simulink model "Powertrain_model_21a"  (R2021a)
settings: Solver=VariableStepAuto  StartTime=0.0  StopTime=1000  RelTol=1e-3
values from neighbouring files (symbols this model uses):
  DR = 5.213    [Sim_script.m]    (also in workspace.mat)
  MaxLimit = [2.1951    294.39 ... (first row only)    [power_distribute_func.m]
  P_CE_idle = 0    [Sim_script.m]    (also in workspace.mat = 1)
  Trans_In = 24.086    [Sim_script.m]    (also in workspace.mat)
  w_CE_idle = 400    [Sim_script.m]    (also in workspace.mat = 32)
undefined symbols (not defined in the file or in its folder): Fuel_con_map, Res_Torque
libraries: pid_lib x2
settings Model: Creator=Sagar Singhal  LastModifiedBy=olsonsao

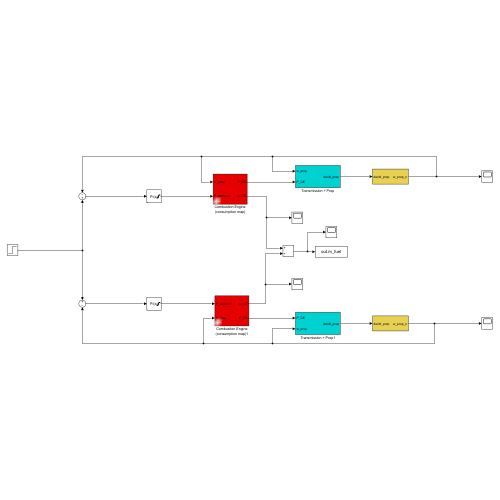
[thumbnail: Simulink's stored preview of the top-level diagram]
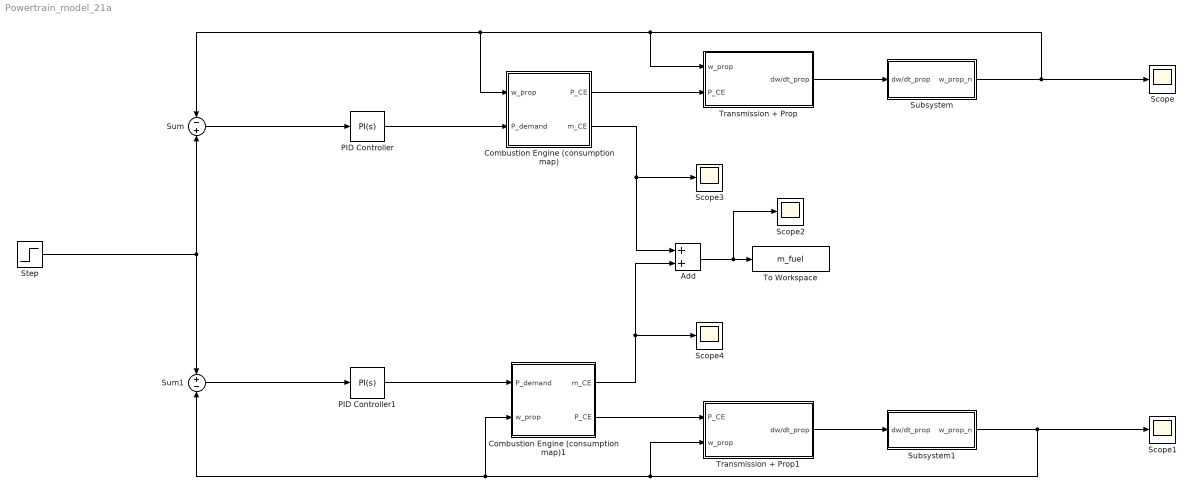
== system Powertrain_model_21a ==
  Add : Sum
  Combustion Engine (consumption map) : Subsystem  Tag=combustion engine  AncestorBlock=|
      | qss_tb_library/Energy Converter/Combustion Engine
      | (consumption map)
  Combustion Engine (consumption map)1 : Subsystem  Tag=combustion engine  AncestorBlock=|
      | qss_tb_library/Energy Converter/Combustion Engine
      | (consumption map)
  PID Controller : pid_lib/PID Controller  Controller=PI  Form=Parallel  TimeDomain=Continuous-time  UseExternalTs=off  SampleTime=-1  IntegratorMethod=Forward Euler  FilterMethod=Forward Euler  ControllerParametersSource=internal  P=6.64458766097002  I=6.35561266010105  D=0  UseFilter=on  N=100  TunerSelectOption=Transfer Function Based (PID Tuner App)  InitialConditionSource=internal  InitialConditionForIntegrator=0  InitialConditionForFilter=0  DifferentiatorICPrevScaledInput=0  ExternalReset=none  TrackingMode=off  Kt=1  LimitOutput=on  SatLimitsSource=internal  UpperSaturationLimit=inf  LowerSaturationLimit=0  LinearizeAsGain=on  AntiWindupMode=none  Kb=1  POutMin=[]  POutMax=[]  IOutMin=[]  IOutMax=[]  DOutMin=[]  DOutMax=[]  NOutMin=[]  NOutMax=[]  SumOutMin=[]  SumOutMax=[]  SaturationOutMin=[]  SaturationOutMax=[]  PParamMin=[]  PParamMax=[]  IParamMin=[]  IParamMax=[]  DParamMin=[]  DParamMax=[]  NParamMin=[]  NParamMax=[]  KbParamMin=[]  KbParamMax=[]  KtParamMin=[]  KtParamMax=[]  KbOutMin=[]  KbOutMax=[]  KtOutMin=[]  KtOutMax=[]  IntegratorOutMin=[]  IntegratorOutMax=[]  FilterOutMin=[]  FilterOutMax=[]  SumI1OutMin=[]  SumI1OutMax=[]  SumI2OutMin=[]  SumI2OutMax=[]  SumI3OutMin=[]  SumI3OutMax=[]  SumI4OutMin=[]  SumI4OutMax=[]  SumDOutMin=[]  SumDOutMax=[]  DifferentiatorOutMin=[]  DifferentiatorOutMax=[]  FilterDiffOutCoefMin=[]  FilterDiffOutCoefMax=[]  ReciprocalOutMin=[]  ReciprocalOutMax=[]  SumDenOutMin=[]  SumDenOutMax=[]  SumNumOutMin=[]  SumNumOutMax=[]  DivideOutMin=[]  DivideOutMax=[]  UdiffTsProdOutMin=[]  UdiffTsProdOutMax=[]  NTsProdOutMin=[]  NTsProdOutMax=[]  UintegralTsProdOutMin=[]  UintegralTsProdOutMax=[]  UngainTsProdOutMin=[]  UngainTsProdOutMax=[]  IntegratorContinuousStateAttributes=''  IntegratorStateMustResolveToSignalObject=off  IntegratorRTWStateStorageClass=Auto  FilterContinuousStateAttributes=''  FilterStateMustResolveToSignalObject=off  FilterRTWStateStorageClass=Auto  ParallelPVariant=InternalParameters  IdealPVariant=Disabled  IVariant=InternalParameters  DVariant=Disabled  IntegratorVariant=Continuous  SatVariant=Enabled  AWVariant=Passthrough  PCopyVariant=Disabled  TRVariant=Disabled  FdbkBlocksVariant=Forward  IdealPFdbkVariant=Disabled  SatFdbkVariant=Disabled  DerivativeFilterVariant=Disabled  NVariant=Disabled  NCopyVariant=Disabled_SignalSpec  FilterICVariant=Disabled  IntegratorICVariant=InternalICs  ExternalResetVariant=Disabled  TRSumVariant=Passthrough  SumFdbkVariant=Disabled  SumVariant=Sum_PI  TsampFilterVariant=InternalTs  TsampNgainVariant=Passthrough  TsampIntegralVariant=Passthrough  ExternalSaturationOutDataTypeStr=Inherit: Same as second input
  PID Controller1 : pid_lib/PID Controller  Controller=PI  Form=Parallel  TimeDomain=Continuous-time  UseExternalTs=off  SampleTime=-1  IntegratorMethod=Forward Euler  FilterMethod=Forward Euler  ControllerParametersSource=internal  P=6.64458766097002  I=6.35561266010105  D=0  UseFilter=on  N=100  TunerSelectOption=Transfer Function Based (PID Tuner App)  InitialConditionSource=internal  InitialConditionForIntegrator=0  InitialConditionForFilter=0  DifferentiatorICPrevScaledInput=0  ExternalReset=none  TrackingMode=off  Kt=1  LimitOutput=on  SatLimitsSource=internal  UpperSaturationLimit=inf  LowerSaturationLimit=0  LinearizeAsGain=on  AntiWindupMode=none  Kb=1  POutMin=[]  POutMax=[]  IOutMin=[]  IOutMax=[]  DOutMin=[]  DOutMax=[]  NOutMin=[]  NOutMax=[]  SumOutMin=[]  SumOutMax=[]  SaturationOutMin=[]  SaturationOutMax=[]  PParamMin=[]  PParamMax=[]  IParamMin=[]  IParamMax=[]  DParamMin=[]  DParamMax=[]  NParamMin=[]  NParamMax=[]  KbParamMin=[]  KbParamMax=[]  KtParamMin=[]  KtParamMax=[]  KbOutMin=[]  KbOutMax=[]  KtOutMin=[]  KtOutMax=[]  IntegratorOutMin=[]  IntegratorOutMax=[]  FilterOutMin=[]  FilterOutMax=[]  SumI1OutMin=[]  SumI1OutMax=[]  SumI2OutMin=[]  SumI2OutMax=[]  SumI3OutMin=[]  SumI3OutMax=[]  SumI4OutMin=[]  SumI4OutMax=[]  SumDOutMin=[]  SumDOutMax=[]  DifferentiatorOutMin=[]  DifferentiatorOutMax=[]  FilterDiffOutCoefMin=[]  FilterDiffOutCoefMax=[]  ReciprocalOutMin=[]  ReciprocalOutMax=[]  SumDenOutMin=[]  SumDenOutMax=[]  SumNumOutMin=[]  SumNumOutMax=[]  DivideOutMin=[]  DivideOutMax=[]  UdiffTsProdOutMin=[]  UdiffTsProdOutMax=[]  NTsProdOutMin=[]  NTsProdOutMax=[]  UintegralTsProdOutMin=[]  UintegralTsProdOutMax=[]  UngainTsProdOutMin=[]  UngainTsProdOutMax=[]  IntegratorContinuousStateAttributes=''  IntegratorStateMustResolveToSignalObject=off  IntegratorRTWStateStorageClass=Auto  FilterContinuousStateAttributes=''  FilterStateMustResolveToSignalObject=off  FilterRTWStateStorageClass=Auto  ParallelPVariant=InternalParameters  IdealPVariant=Disabled  IVariant=InternalParameters  DVariant=Disabled  IntegratorVariant=Continuous  SatVariant=Enabled  AWVariant=Passthrough  PCopyVariant=Disabled  TRVariant=Disabled  FdbkBlocksVariant=Forward  IdealPFdbkVariant=Disabled  SatFdbkVariant=Disabled  DerivativeFilterVariant=Disabled  NVariant=Disabled  NCopyVariant=Disabled_SignalSpec  FilterICVariant=Disabled  IntegratorICVariant=InternalICs  ExternalResetVariant=Disabled  TRSumVariant=Passthrough  SumFdbkVariant=Disabled  SumVariant=Sum_PI  TsampFilterVariant=InternalTs  TsampNgainVariant=Passthrough  TsampIntegralVariant=Passthrough  ExternalSaturationOutDataTypeStr=Inherit: Same as second input
  Scope{,1..4} (5 alike) : Scope
  Step : Step  Time=500  Before=100  After=400  SampleTime=0
  Subsystem : Subsystem
  Subsystem1 : Subsystem
  Sum : Sum  Inputs=-|+
  Sum1 : Sum  Inputs=+|-
  To Workspace : ToWorkspace  VariableName=m_fuel  SaveFormat=Timeseries  SampleTime=-1
  Transmission + Prop : Subsystem
  Transmission + Prop1 : Subsystem
  wires:
  Combustion Engine (consumption map)/1(P_CE) -> Transmission + Prop/2(P_CE)
  Transmission + Prop/1(dw/dt_prop) -> Subsystem/1(dw/dt_prop)
  Combustion Engine (consumption map)/2(m_CE) -> Scope3/1, Add/1
  Subsystem/1(w_prop_n) -> Scope/1, Transmission + Prop/1(w_prop), Combustion Engine (consumption map)/1(w_prop), Sum/1
  Sum/1 -> PID Controller/1
  PID Controller/1 -> Combustion Engine (consumption map)/2(P_demand)
  PID Controller1/1 -> Combustion Engine (consumption map)1/1(P_demand)
  Sum1/1 -> PID Controller1/1
  Combustion Engine (consumption map)1/2(P_CE) -> Transmission + Prop1/1(P_CE)
  Subsystem1/1(w_prop_n) -> Scope1/1, Transmission + Prop1/2(w_prop), Sum1/2, Combustion Engine (consumption map)1/2(w_prop)
  Transmission + Prop1/1(dw/dt_prop) -> Subsystem1/1(dw/dt_prop)
  Combustion Engine (consumption map)1/1(m_CE) -> Scope4/1, Add/2
  Step/1 -> Sum/2, Sum1/1
  Add/1 -> To Workspace/1, Scope2/1

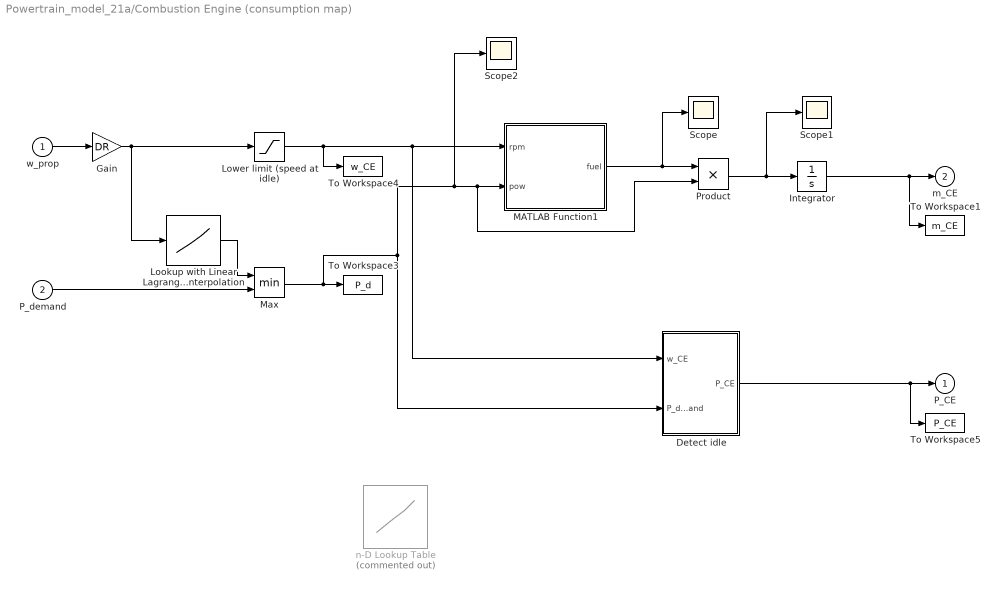
== system Powertrain_model_21a/Combustion Engine (consumption map) ==
  w_prop : Inport
  P_demand : Inport  Port=2
  Detect idle : Subsystem
  Gain : Gain  Gain=DR
  Integrator : Integrator
  Lookup with Linear Lagrange Interpolation : Lookup_n-D  NumberOfTableDimensions=1  BreakpointsForDimension1=MaxLimit.('RPM')  Table=MaxLimit.('Pow_kW_')  InterpMethod=Linear Lagrange  InternalRulePriority=Speed  RndMeth=Simplest  InputSameDT=on
  Lower limit (speed at idle) : Saturate  UpperLimit=inf  LowerLimit=w_CE_idle
  MATLAB Function1 : MATLAB Function  TreatAsAtomicUnit=on
  Max : MinMax  Inputs=2
  Product : Product
  Scope : Scope
  Scope1 : Scope
  Scope2 : Scope
  To Workspace1 : ToWorkspace  VariableName=m_CE  SampleTime=-1
  To Workspace3 : ToWorkspace  VariableName=P_d  SampleTime=-1
  To Workspace4 : ToWorkspace  VariableName=w_CE  SampleTime=-1
  To Workspace5 : ToWorkspace  VariableName=P_CE  SampleTime=-1
  n-D Lookup Table : Lookup_n-D  Commented=on  LookupTableObject=''  BreakpointsForDimension1=Fuel_con_map.('RPM')  BreakpointsForDimension2=Fuel_con_map.('Power(kW)')  BreakpointsForDimension3=[5, 7]  BreakpointsForDimension1FirstPoint=10  BreakpointsForDimension2FirstPoint=10  BreakpointsForDimension1Spacing=12  BreakpointsForDimension2Spacing=12  IndexSearchMethod=Evenly spaced points  Table=Fuel_con_map.('Fuel(g/KWh)')  InterpMethod=Cubic spline  ExtrapMethod=Cubic spline  DiagnosticForOutOfRangeInput=Error  InternalRulePriority=Speed  RndMeth=Simplest  InputSameDT=on
      settings: InputPortMap=u0,u1
  P_CE : Outport  InitialOutput=0
  m_CE : Outport  Port=2  InitialOutput=0
  wires:
  Integrator/1 -> To Workspace1/1, m_CE/1
  w_prop/1 -> Gain/1
  Detect idle/1(P_CE) -> To Workspace5/1, P_CE/1
  Lookup with Linear Lagrange Interpolation/1 -> Max/1
  Gain/1 -> Lookup with Linear Lagrange Interpolation/1, Lower limit (speed at idle)/1
  P_demand/1 -> Max/2
  MATLAB Function1/1(fuel) -> Scope/1, Product/1
  Lower limit (speed at idle)/1 -> To Workspace4/1, MATLAB Function1/1(rpm), Detect idle/1(w_CE)
  Product/1 -> Scope1/1, Integrator/1
  Max/1 -> Scope2/1, Product/2, MATLAB Function1/2(pow), Detect idle/2(P_demand), To Workspace3/1

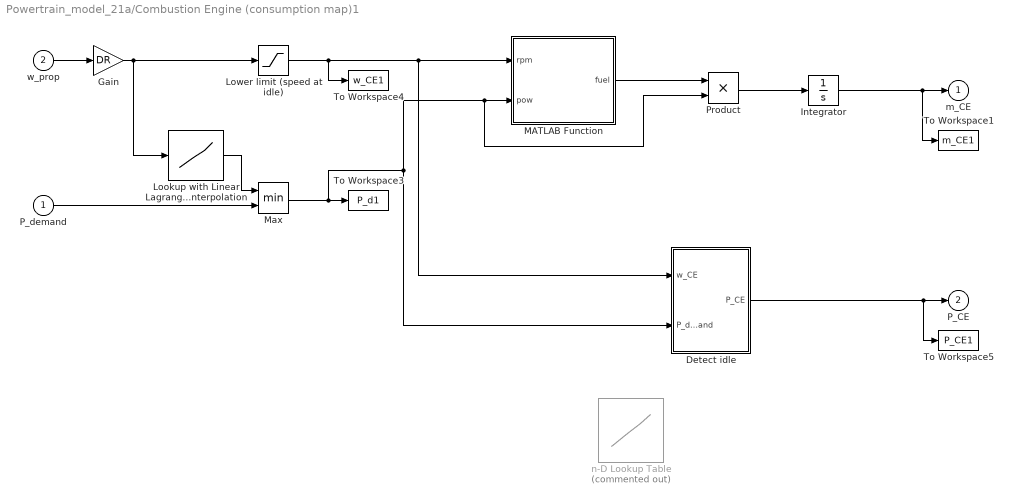
== system Powertrain_model_21a/Combustion Engine (consumption map)1 ==
  P_demand : Inport
  w_prop : Inport  Port=2
  Detect idle : Subsystem
  Gain : Gain  Gain=DR
  Integrator : Integrator
  Lookup with Linear Lagrange Interpolation : Lookup_n-D  NumberOfTableDimensions=1  BreakpointsForDimension1=MaxLimit.('RPM')  Table=MaxLimit.('Pow_kW_')  InterpMethod=Linear Lagrange  InternalRulePriority=Speed  RndMeth=Simplest  InputSameDT=on
  Lower limit (speed at idle) : Saturate  UpperLimit=inf  LowerLimit=w_CE_idle
  MATLAB Function : MATLAB Function  TreatAsAtomicUnit=on
  Max : MinMax  Inputs=2
  Product : Product
  To Workspace1 : ToWorkspace  VariableName=m_CE1  SampleTime=-1
  To Workspace3 : ToWorkspace  VariableName=P_d1  SampleTime=-1
  To Workspace4 : ToWorkspace  VariableName=w_CE1  SampleTime=-1
  To Workspace5 : ToWorkspace  VariableName=P_CE1  SampleTime=-1
  n-D Lookup Table : Lookup_n-D  Commented=on  LookupTableObject=''  BreakpointsForDimension1=Fuel_con_map.('RPM')  BreakpointsForDimension2=Fuel_con_map.('Power(kW)')  BreakpointsForDimension3=[5, 7]  BreakpointsForDimension1FirstPoint=10  BreakpointsForDimension2FirstPoint=10  BreakpointsForDimension1Spacing=12  BreakpointsForDimension2Spacing=12  IndexSearchMethod=Evenly spaced points  Table=Fuel_con_map.('Fuel(g/KWh)')  InterpMethod=Cubic spline  ExtrapMethod=Cubic spline  DiagnosticForOutOfRangeInput=Error  InternalRulePriority=Speed  RndMeth=Simplest  InputSameDT=on
      settings: InputPortMap=u0,u1
  m_CE : Outport  InitialOutput=0
  P_CE : Outport  Port=2  InitialOutput=0
  wires:
  Max/1 -> Product/2, MATLAB Function/2(pow), Detect idle/2(P_demand), To Workspace3/1
  Product/1 -> Integrator/1
  w_prop/1 -> Gain/1
  Lower limit (speed at idle)/1 -> To Workspace4/1, Detect idle/1(w_CE), MATLAB Function/1(rpm)
  Detect idle/1(P_CE) -> To Workspace5/1, P_CE/1
  Lookup with Linear Lagrange Interpolation/1 -> Max/1
  Gain/1 -> Lookup with Linear Lagrange Interpolation/1, Lower limit (speed at idle)/1
  P_demand/1 -> Max/2
  MATLAB Function/1(fuel) -> Product/1
  Integrator/1 -> To Workspace1/1, m_CE/1

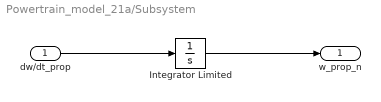
== system Powertrain_model_21a/Subsystem ==
  dw/dt_prop : Inport
  Integrator Limited : Integrator  InitialCondition=100  UpperSaturationLimit=1  LowerSaturationLimit=0
  w_prop_n : Outport
  wires:
  dw/dt_prop/1 -> Integrator Limited/1
  Integrator Limited/1 -> w_prop_n/1

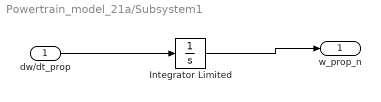
== system Powertrain_model_21a/Subsystem1 ==
  dw/dt_prop : Inport
  Integrator Limited : Integrator  InitialCondition=100  UpperSaturationLimit=1  LowerSaturationLimit=0
  w_prop_n : Outport
  wires:
  dw/dt_prop/1 -> Integrator Limited/1
  Integrator Limited/1 -> w_prop_n/1

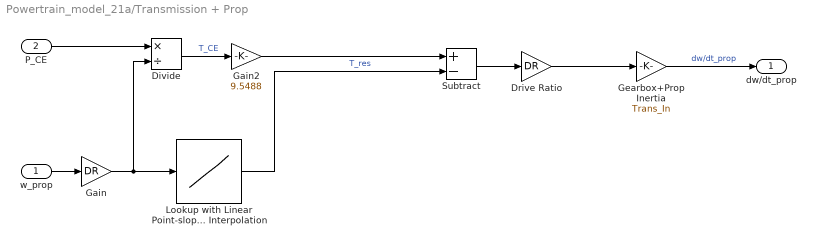
== system Powertrain_model_21a/Transmission + Prop ==
  w_prop : Inport
  P_CE : Inport  Port=2
  Divide : Product  Inputs=*/
  Drive Ratio : Gain  Gain=DR
  Gain : Gain  Gain=DR
  Gain2 : Gain  Gain=9.5488
  Gearbox+Prop Inertia : Gain  Gain=Trans_In
  Lookup with Linear Point-slope Interpolation : Lookup_n-D  NumberOfTableDimensions=1  BreakpointsForDimension1=Res_Torque.('RPMEngine')  Table=Res_Torque.('TorqueNM')  InternalRulePriority=Speed  RndMeth=Simplest  InputSameDT=on
  Subtract : Sum  Inputs=+-
  dw/dt_prop : Outport
  wires:
  Lookup with Linear Point-slope Interpolation/1 -> Subtract/2  "T_res"
  P_CE/1 -> Divide/1
  Subtract/1 -> Drive Ratio/1
  Gearbox+Prop Inertia/1 -> dw/dt_prop/1  "dw/dt_prop"
  w_prop/1 -> Gain/1
  Drive Ratio/1 -> Gearbox+Prop Inertia/1
  Divide/1 -> Gain2/1  "T_CE"
  Gain/1 -> Divide/2, Lookup with Linear Point-slope Interpolation/1
  Gain2/1 -> Subtract/1

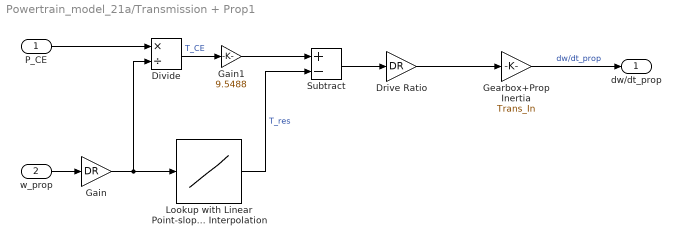
== system Powertrain_model_21a/Transmission + Prop1 ==
  P_CE : Inport
  w_prop : Inport  Port=2
  Divide : Product  Inputs=*/
  Drive Ratio : Gain  Gain=DR
  Gain : Gain  Gain=DR
  Gain1 : Gain  Gain=9.5488
  Gearbox+Prop Inertia : Gain  Gain=Trans_In
  Lookup with Linear Point-slope Interpolation : Lookup_n-D  NumberOfTableDimensions=1  BreakpointsForDimension1=Res_Torque.('RPMEngine')  Table=Res_Torque.('TorqueNM')  InternalRulePriority=Speed  RndMeth=Simplest  InputSameDT=on
  Subtract : Sum  Inputs=+-
  dw/dt_prop : Outport
  wires:
  Lookup with Linear Point-slope Interpolation/1 -> Subtract/2  "T_res"
  P_CE/1 -> Divide/1
  Subtract/1 -> Drive Ratio/1
  Gearbox+Prop Inertia/1 -> dw/dt_prop/1  "dw/dt_prop"
  w_prop/1 -> Gain/1
  Drive Ratio/1 -> Gearbox+Prop Inertia/1
  Divide/1 -> Gain1/1  "T_CE"
  Gain/1 -> Divide/2, Lookup with Linear Point-slope Interpolation/1
  Gain1/1 -> Subtract/1

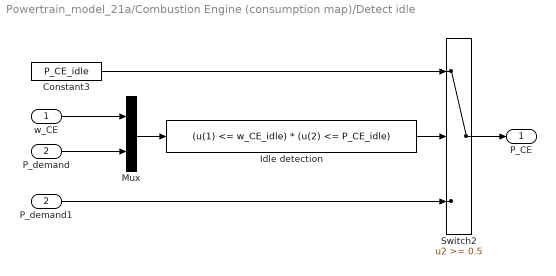
== system Powertrain_model_21a/Combustion Engine (consumption map)/Detect idle ==
  w_CE : Inport
  P_demand : Inport  Port=2
  Constant3 : Constant  Value=P_CE_idle
  Idle detection : Fcn  Expr=(u(1) <= w_CE_idle) * (u(2) <= P_CE_idle)
  Mux : Mux  Inputs=2
  P_demand1 : InportShadow  Port=2
  Switch2 : Switch  Threshold=0.5  SaturateOnIntegerOverflow=on  InputSameDT=on
  P_CE : Outport  InitialOutput=0
  wires:
  Constant3/1 -> Switch2/1
  Switch2/1 -> P_CE/1
  P_demand1/1 -> Switch2/3
  Idle detection/1 -> Switch2/2
  w_CE/1 -> Mux/1
  P_demand/1 -> Mux/2
  Mux/1 -> Idle detection/1

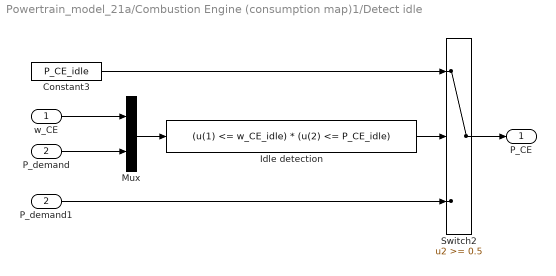
== system Powertrain_model_21a/Combustion Engine (consumption map)1/Detect idle ==
  w_CE : Inport
  P_demand : Inport  Port=2
  Constant3 : Constant  Value=P_CE_idle
  Idle detection : Fcn  Expr=(u(1) <= w_CE_idle) * (u(2) <= P_CE_idle)
  Mux : Mux  Inputs=2
  P_demand1 : InportShadow  Port=2
  Switch2 : Switch  Threshold=0.5  SaturateOnIntegerOverflow=on  InputSameDT=on
  P_CE : Outport  InitialOutput=0
  wires:
  Constant3/1 -> Switch2/1
  Switch2/1 -> P_CE/1
  P_demand1/1 -> Switch2/3
  Idle detection/1 -> Switch2/2
  w_CE/1 -> Mux/1
  P_demand/1 -> Mux/2
  Mux/1 -> Idle detection/1

== matlab function Powertrain_model_21a/Combustion Engine (consumption map)/MATLAB Function1 ==
  data: rpm input; fuel output; pow input
function fuel   = fuel_con_map(rpm,pow)
x = (rpm-1180)/409.7;
y = (pow-876.1)/438.6;
p00 =         203;
p10 =      0.9394;
p01 =      -8.327;
p20 =       1.894;
p11 =     -0.7168;
p02 =       1.321;
p30 =      0.2621;
p21 =       1.482;
p12 =       5.529;
p03 =      -2.619;
p40 =      0.9252;
p31 =      -3.236;
p22 =       3.413;
p13 =      -2.546;
p04 =        2.97;
p50 =     -0.1717;
p41 =       1.492;
p32 =      -2.908;
p23 =      0.2029;
p14 =      0.4508;
p05 =     -0.7973;
fuel = p00 + p10*x + p01*y + p20*x^2 + p11*x*y + p02*y^2 + p30*x^3 + p21*x^2*y ...
         + p12*x*y^2 + p03*y^3 + p40*x^4 + p31*x^3*y + p22*x^2*y^2 ...
         + p13*x*y^3 + p04*y^4 + p50*x^5 + p41*x^4*y + p32*x^3*y^2 ...
          + p23*x^2*y^3 + p14*x*y^4 + p05*y^5;
end

== matlab function Powertrain_model_21a/Combustion Engine (consumption map)1/MATLAB Function ==
  data: rpm input; fuel output; pow input
function fuel  = fuel_con_map(rpm,pow)
x = (rpm-1180)/409.7;
y = (pow-876.1)/438.6;
p00 =         203;
p10 =      0.9394;
p01 =      -8.327;
p20 =       1.894;
p11 =     -0.7168;
p02 =       1.321;
p30 =      0.2621;
p21 =       1.482;
p12 =       5.529;
p03 =      -2.619;
p40 =      0.9252;
p31 =      -3.236;
p22 =       3.413;
p13 =      -2.546;
p04 =        2.97;
p50 =     -0.1717;
p41 =       1.492;
p32 =      -2.908;
p23 =      0.2029;
p14 =      0.4508;
p05 =     -0.7973;
fuel = p00 + p10*x + p01*y + p20*x^2 + p11*x*y + p02*y^2 + p30*x^3 + p21*x^2*y ...
         + p12*x*y^2 + p03*y^3 + p40*x^4 + p31*x^3*y + p22*x^2*y^2 ...
         + p13*x*y^3 + p04*y^4 + p50*x^5 + p41*x^4*y + p32*x^3*y^2 ...
          + p23*x^2*y^3 + p14*x*y^4 + p05*y^5;
end
